simulink model "prima_simulazione_2021b"  (R2021b)
settings: Solver=VariableStepAuto  StartTime=0.0  StopTime=T_sim  RelTol=1e-3
values from neighbouring files (symbols this model uses):
  k = 1    [main.m]
  tau = 2    [main.m]
undefined symbols (not defined in the file or in its folder): h_max, kg_to_m, livello_0, m_to_kg, step_liq, step_time
settings Model: Creator=pmong  LastModifiedBy=pmong
settings DebuggingCC: UnconnectedInputMsg=none  UnconnectedOutputMsg=none  UnconnectedLineMsg=none
settings ModelReferenceCC: EnableRefExpFcnMdlSchedulingChecks=off
settings RTWCC: DLArmComputeVersion=20.02.1

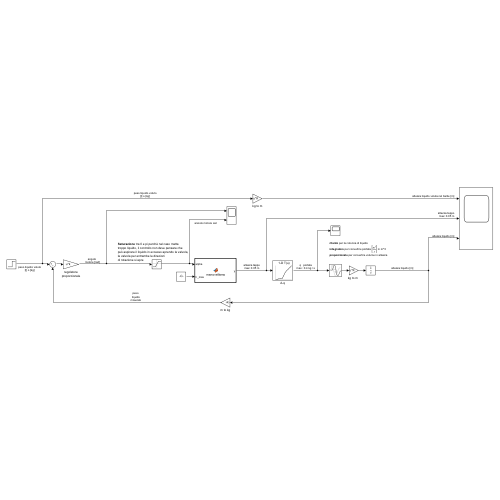
[thumbnail: Simulink's stored preview of the top-level diagram]
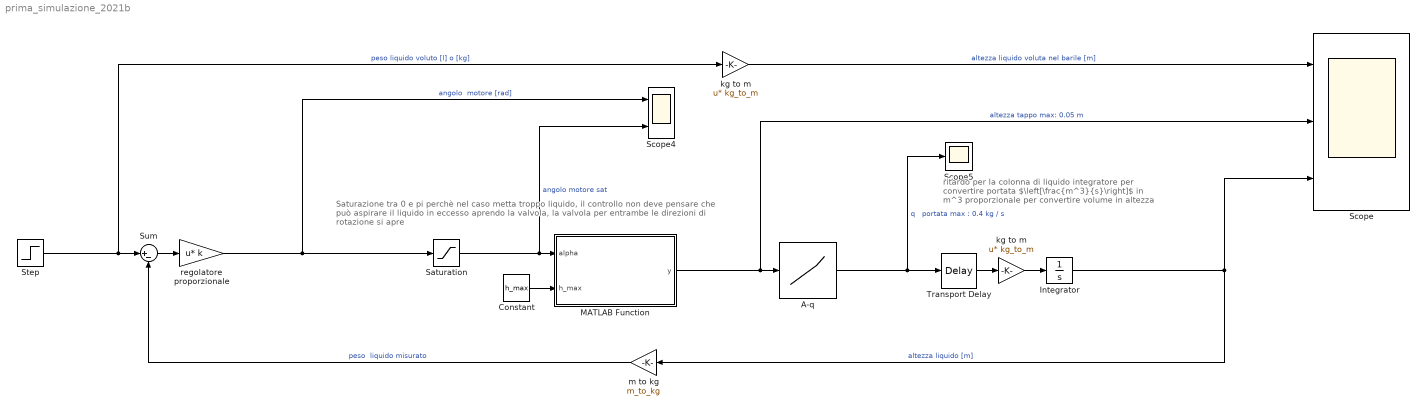
== system prima_simulazione_2021b ==
  note: Saturazione tra 0 e pi perchè nel caso metta
      | troppo liquido, il controllo non deve pensare che
      | può aspirare il liquido in eccesso aprendo la valvola,
      | la valvola per entrambe le direzioni
      | di rotazione si apre
  note: ritardo per la colonna di liquido
      | integratore per convertire portata $\left[\frac{m^3}{s}\right]$ in m^3
      | proporzionale per convertire volume in altezza
  A-q : Lookup_n-D  NumberOfTableDimensions=1  BreakpointsForDimension1=[0 0.005 0.01 0.015 0.02 0.025 0.03 0.035 0.04 0.045 0.05]  Table=[0 0.005 0.01 0.015 0.02 0.1 0.2 0.25 0.3 0.35 0.4]  InternalRulePriority=Speed  RndMeth=Simplest  InputSameDT=on
  Constant : Constant  Value=h_max
  Integrator : Integrator
  MATLAB Function : MATLAB Function  TreatAsAtomicUnit=on
  Saturation : Saturate  UpperLimit=pi  LowerLimit=0
  Scope : Scope  NumInputPorts=3
  Scope4 : Scope  NumInputPorts=2
  Scope5 : Scope
  Step : Step  Time=step_time  After=step_liq  SampleTime=0
  Sum : Sum  Inputs=|+-
  Transport Delay : TransportDelay  DelayTime=tau  InitialOutput=livello_0
  kg to m : Gain  Gain=kg_to_m  Multiplication=Matrix(u*K)
  "kg to m  " : Gain  Gain=kg_to_m  Multiplication=Matrix(u*K)
  m to kg : Gain  Gain=m_to_kg
  regolatore proporzionale : Gain  Gain=k  Multiplication=Matrix(u*K)
  wires:
  Step/1 -> Sum/1, kg to m/1  "peso liquido voluto [l] o [kg]"
  Sum/1 -> regolatore proporzionale/1
  MATLAB Function/1(y) -> A-q/1, Scope/2  "altezza tappo max: 0.05 m"
  A-q/1 -> Transport Delay/1, Scope5/1  "q   portata max : 0.4 kg / s"
  m to kg/1 -> Sum/2  "peso  liquido misurato"
  Integrator/1 -> m to kg/1, Scope/3  "altezza liquido [m]"
  regolatore proporzionale/1 -> Saturation/1, Scope4/1  "angolo  motore [rad]"
  Constant/1 -> MATLAB Function/2(h_max)
  Saturation/1 -> MATLAB Function/1(alpha), Scope4/2  "angolo motore sat"
  kg to m/1 -> Scope/1  "altezza liquido voluta nel barile [m]"
  Transport Delay/1 -> "kg to m  "/1
  "kg to m  "/1 -> Integrator/1

== matlab function prima_simulazione_2021b/MATLAB Function ==
  data: alpha input; y output; h_max input

function y = manovellismo(alpha, h_max)
y = h_max * 0.5 *(1-cos(alpha));
end
